simulink model "combinedmodels"  (R2022b)
settings: Solver=VariableStepAuto  StartTime=0.0  StopTime=3600  RelTol=1e-3
libraries: sh_lib x46, spsThreePhaseVIMeasurementLib x36, spsThreePhaseSeriesRLCLoadLib x32, spsThreePhaseSeriesRLCBranchLib x32, fl_lib x27, nesl_utility x25, spsCurrentVoltageSimscapeInterfacegndLib x6, ee_lib x3, spsGroundLib x3, spsPower3phPhasorLib x3, SignalEditorBlockLib x3, spsThreePhaseParallelRLCBranchLib x3
(part 3 of 3)

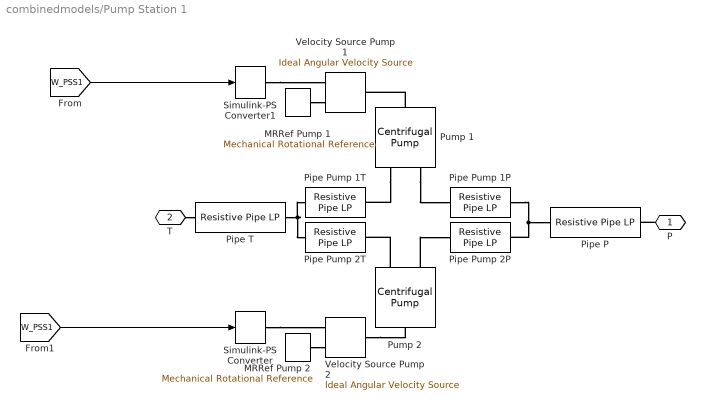
== system combinedmodels/Pump Station 1 ==
  MRRef Pump 1 : fl_lib/Mechanical/Rotational Elements/Mechanical Rotational Reference
  MRRef Pump 2 : fl_lib/Mechanical/Rotational Elements/Mechanical Rotational Reference
  Pipe P : sh_lib/Low-Pressure Blocks/Resistive Pipe LP  cs_type=1  d_in=station_1.pipe_diameter mm  area=1e-04 m^2  D_h=0.0112 m  s_factor=64  length=station_1.pipe_length_3 m  length_ad=1 m  roughness=0.005 mm  Re_lam=2e+03  Re_turb=4e+03  elevation_A=station_1.elevation m  elevation_B=station_1.elevation m  g=9.80665 m/s^2  pressure_drop_specify=off  pressure_drop_priority=None  pressure_drop=0 Pa  pressure_drop_nominal_specify=off  pressure_drop_nominal_unit=Pa  pressure_drop_nominal_value=1  flow_rate_specify=off  flow_rate_priority=None  flow_rate=0 m^3/s  flow_rate_nominal_specify=off  flow_rate_nominal_unit=m^3/s  flow_rate_nominal_value=1
      settings: InternalSimscapePortConfiguration="{\"Bottom\":[],\"Left\":[{\"id\":\"A\",\"label\":\"A\",\"type\":\"foundation.hydraulic.hydraulic\"}],\"Right\":[{\"id\":\"B\",\"label\":\"B\",\"type\":\"foundation.hydraulic.hydraulic\"}],\"Top\":[]}"
  Pipe Pump 1P : sh_lib/Low-Pressure Blocks/Resistive Pipe LP  cs_type=1  d_in=station_1.pipe_diameter mm  area=1e-04 m^2  D_h=0.0112 m  s_factor=64  length=station_1.pipe_length_2 m  length_ad=1 m  roughness=0.005 mm  Re_lam=2e+03  Re_turb=4e+03  elevation_A=station_1.elevation m  elevation_B=station_1.elevation m  g=9.80665 m/s^2  pressure_drop_specify=off  pressure_drop_priority=None  pressure_drop=0 Pa  pressure_drop_nominal_specify=off  pressure_drop_nominal_unit=Pa  pressure_drop_nominal_value=1  flow_rate_specify=off  flow_rate_priority=None  flow_rate=0 m^3/s  flow_rate_nominal_specify=off  flow_rate_nominal_unit=m^3/s  flow_rate_nominal_value=1
      settings: InternalSimscapePortConfiguration="{\"Bottom\":[],\"Left\":[{\"id\":\"A\",\"label\":\"A\",\"type\":\"foundation.hydraulic.hydraulic\"}],\"Right\":[{\"id\":\"B\",\"label\":\"B\",\"type\":\"foundation.hydraulic.hydraulic\"}],\"Top\":[]}"
  Pipe Pump 1T : sh_lib/Low-Pressure Blocks/Resistive Pipe LP  cs_type=1  d_in=station_1.pipe_diameter mm  area=1e-04 m^2  D_h=0.0112 m  s_factor=64  length=station_1.pipe_length_2 m  length_ad=1 m  roughness=0.005 mm  Re_lam=2e+03  Re_turb=4e+03  elevation_A=station_1.elevation m  elevation_B=station_1.elevation m  g=9.80665 m/s^2  pressure_drop_specify=off  pressure_drop_priority=None  pressure_drop=0 Pa  pressure_drop_nominal_specify=off  pressure_drop_nominal_unit=Pa  pressure_drop_nominal_value=1  flow_rate_specify=off  flow_rate_priority=None  flow_rate=0 m^3/s  flow_rate_nominal_specify=off  flow_rate_nominal_unit=m^3/s  flow_rate_nominal_value=1
      settings: InternalSimscapePortConfiguration="{\"Bottom\":[],\"Left\":[{\"id\":\"A\",\"label\":\"A\",\"type\":\"foundation.hydraulic.hydraulic\"}],\"Right\":[{\"id\":\"B\",\"label\":\"B\",\"type\":\"foundation.hydraulic.hydraulic\"}],\"Top\":[]}"
  Pipe Pump 2P : sh_lib/Low-Pressure Blocks/Resistive Pipe LP  cs_type=1  d_in=station_1.pipe_diameter mm  area=1e-04 m^2  D_h=0.0112 m  s_factor=64  length=station_1.pipe_length_2 m  length_ad=1 m  roughness=0.005 mm  Re_lam=2e+03  Re_turb=4e+03  elevation_A=station_1.elevation m  elevation_B=station_1.elevation m  g=9.80665 m/s^2  pressure_drop_specify=off  pressure_drop_priority=None  pressure_drop=0 Pa  pressure_drop_nominal_specify=off  pressure_drop_nominal_unit=Pa  pressure_drop_nominal_value=1  flow_rate_specify=off  flow_rate_priority=None  flow_rate=0 m^3/s  flow_rate_nominal_specify=off  flow_rate_nominal_unit=m^3/s  flow_rate_nominal_value=1
      settings: InternalSimscapePortConfiguration="{\"Bottom\":[],\"Left\":[{\"id\":\"A\",\"label\":\"A\",\"type\":\"foundation.hydraulic.hydraulic\"}],\"Right\":[{\"id\":\"B\",\"label\":\"B\",\"type\":\"foundation.hydraulic.hydraulic\"}],\"Top\":[]}"
  Pipe Pump 2T : sh_lib/Low-Pressure Blocks/Resistive Pipe LP  cs_type=1  d_in=station_1.pipe_diameter mm  area=1e-04 m^2  D_h=0.0112 m  s_factor=64  length=station_1.pipe_length_2 m  length_ad=1 m  roughness=0.005 mm  Re_lam=2e+03  Re_turb=4e+03  elevation_A=station_1.elevation m  elevation_B=station_1.elevation m  g=9.80665 m/s^2  pressure_drop_specify=off  pressure_drop_priority=None  pressure_drop=0 Pa  pressure_drop_nominal_specify=off  pressure_drop_nominal_unit=Pa  pressure_drop_nominal_value=1  flow_rate_specify=off  flow_rate_priority=None  flow_rate=0 m^3/s  flow_rate_nominal_specify=off  flow_rate_nominal_unit=m^3/s  flow_rate_nominal_value=1
      settings: InternalSimscapePortConfiguration="{\"Bottom\":[],\"Left\":[{\"id\":\"A\",\"label\":\"A\",\"type\":\"foundation.hydraulic.hydraulic\"}],\"Right\":[{\"id\":\"B\",\"label\":\"B\",\"type\":\"foundation.hydraulic.hydraulic\"}],\"Top\":[]}"
  Pipe T : sh_lib/Low-Pressure Blocks/Resistive Pipe LP  cs_type=1  d_in=station_1.pipe_diameter mm  area=1e-04 m^2  D_h=0.0112 m  s_factor=64  length=station_1.pipe_length_1 m  length_ad=1 m  roughness=0.005 mm  Re_lam=2e+03  Re_turb=4e+03  elevation_A=station_1.elevation m  elevation_B=station_1.elevation m  g=9.80665 m/s^2  pressure_drop_specify=off  pressure_drop_priority=None  pressure_drop=0 Pa  pressure_drop_nominal_specify=off  pressure_drop_nominal_unit=Pa  pressure_drop_nominal_value=1  flow_rate_specify=off  flow_rate_priority=None  flow_rate=0 m^3/s  flow_rate_nominal_specify=off  flow_rate_nominal_unit=m^3/s  flow_rate_nominal_value=1
      settings: InternalSimscapePortConfiguration="{\"Bottom\":[],\"Left\":[{\"id\":\"A\",\"label\":\"A\",\"type\":\"foundation.hydraulic.hydraulic\"}],\"Right\":[{\"id\":\"B\",\"label\":\"B\",\"type\":\"foundation.hydraulic.hydraulic\"}],\"Top\":[]}"
  Pump 1 : sh_lib/Pumps and Motors/Centrifugal Pump  mdl_type=2  c_1=326.8 Pa/(kg/m^3)  c_2=3.104e+04 Pa*s/kg  c_3=1.097e+07 Pa*s^2/(kg*m^3)  c_4=2.136e+05 Pa*s^2/(kg*m^3)  c_f=0.8  design_del=130 lpm  ref_velocity=2.5e+03 rpm  ref_density=1000 kg/m^3  leak_resistance=1e+8 Pa/(m^3/s)  T_const=0.1 N*m  trq_press_coeff=1e-6 N*m/Pa  pump_del_1D=pump_1.Q m^3/s  press_diff_1D=pump_1.P bar  pump_del_power_1D=pump_1.Q m^3/s  power_1D=pump_1.N W  pump_vel_2D="[  3.2e+03 3.3e+03 3.4e+03 3.5e+03 ] rpm"  pump_del_2D="[  0 50 100 150 200 250 300 350 ] lpm"  press_diff_2D="[  8.3 8.8 9.3 9.9 ; 7.8 8.3 8.8 9.4 ; 7.2 7.6 8.2 8.7 ; 6.5 7 7.5 8 ; 5.6 6.1 6.6 7.1 ; 4.7 5.2 5.7 6.2 ; 3.4 4 4.4 4.9 ; 2.3 2.7 3.4 3.6 ; ] bar"  pump_del_power_2D="[  0 50 100 150 200 250 300 350 ] lpm"  power_2D="[  1.223e+03 1.341e+03 1.467e+03 1.6e+03 ; 1.414e+03 1.551e+03 1.696e+03 1.85e+03 ; 1.636e+03 1.794e+03 1.962e+03 2.14e+03 ; 1.941e+03 2.129e+03 2.326e+03 2.54e+03 ; 2.224e+03 2.439e+03 2.66e+03 2.91e+03 ; 2.453e+03 2.691e+03 2.947e+03 3.21e+03 ; 2.757e+03 3.024e+03 3.307e+03 3.608e+03 ; 2.945e+03 3.23e+03 3.533e+03 3.854e+03 ; ] W"  omega_threshold=1e-9 rad/s  interp_method=2  extrap_method=1
      settings: InternalSimscapePortConfiguration="{\"Bottom\":[],\"Left\":[{\"id\":\"S\",\"label\":\"S\",\"type\":\"foundation.mechanical.rotational.rotational\"}],\"Right\":[{\"id\":\"P\",\"label\":\"P\",\"type\":\"foundation.hydraulic.hydraulic\"},{\"id\":\"T\",\"label\":\"T\",\"type\":\"foundation.hydraulic.hydraulic\"}],\"Top\":[]}"
  Pump 2 : sh_lib/Pumps and Motors/Centrifugal Pump  mdl_type=2  c_1=326.8 Pa/(kg/m^3)  c_2=3.104e+04 Pa*s/kg  c_3=1.097e+07 Pa*s^2/(kg*m^3)  c_4=2.136e+05 Pa*s^2/(kg*m^3)  c_f=0.8  design_del=130 lpm  ref_velocity=2.5e+03 rpm  ref_density=1000 kg/m^3  leak_resistance=1e+8 Pa/(m^3/s)  T_const=0.1 N*m  trq_press_coeff=1e-6 N*m/Pa  pump_del_1D=pump_1.Q m^3/s  press_diff_1D=pump_1.P bar  pump_del_power_1D=pump_1.Q m^3/s  power_1D=pump_1.N W  pump_vel_2D="[  3.2e+03 3.3e+03 3.4e+03 3.5e+03 ] rpm"  pump_del_2D="[  0 50 100 150 200 250 300 350 ] lpm"  press_diff_2D="[  8.3 8.8 9.3 9.9 ; 7.8 8.3 8.8 9.4 ; 7.2 7.6 8.2 8.7 ; 6.5 7 7.5 8 ; 5.6 6.1 6.6 7.1 ; 4.7 5.2 5.7 6.2 ; 3.4 4 4.4 4.9 ; 2.3 2.7 3.4 3.6 ; ] bar"  pump_del_power_2D="[  0 50 100 150 200 250 300 350 ] lpm"  power_2D="[  1.223e+03 1.341e+03 1.467e+03 1.6e+03 ; 1.414e+03 1.551e+03 1.696e+03 1.85e+03 ; 1.636e+03 1.794e+03 1.962e+03 2.14e+03 ; 1.941e+03 2.129e+03 2.326e+03 2.54e+03 ; 2.224e+03 2.439e+03 2.66e+03 2.91e+03 ; 2.453e+03 2.691e+03 2.947e+03 3.21e+03 ; 2.757e+03 3.024e+03 3.307e+03 3.608e+03 ; 2.945e+03 3.23e+03 3.533e+03 3.854e+03 ; ] W"  omega_threshold=1e-9 rad/s  interp_method=2  extrap_method=1
      settings: InternalSimscapePortConfiguration="{\"Bottom\":[],\"Left\":[{\"id\":\"S\",\"label\":\"S\",\"type\":\"foundation.mechanical.rotational.rotational\"}],\"Right\":[{\"id\":\"P\",\"label\":\"P\",\"type\":\"foundation.hydraulic.hydraulic\"},{\"id\":\"T\",\"label\":\"T\",\"type\":\"foundation.hydraulic.hydraulic\"}],\"Top\":[]}"
  Simulink-PS Converter : nesl_utility/Simulink-PS Converter  PhysicalDomain=network_engine_domain  SubClassName=ps_input  LeftPortType=input  RightPortType=output  PseudoPeriodic=off  Frequencies=[]  NoiseDistribution=none  NoiseParameters=[]  Unit=rpm  AffineConversion=off  FilteringAndDerivatives=zero  SimscapeFilterOrder=1  InputFilterTimeConstant=.001  UdotUserProvided=0
  Simulink-PS Converter1 : nesl_utility/Simulink-PS Converter  PhysicalDomain=network_engine_domain  SubClassName=ps_input  LeftPortType=input  RightPortType=output  PseudoPeriodic=off  Frequencies=[]  NoiseDistribution=none  NoiseParameters=[]  Unit=rpm  AffineConversion=off  FilteringAndDerivatives=zero  SimscapeFilterOrder=1  InputFilterTimeConstant=.001  UdotUserProvided=0
  Velocity Source Pump 1 : fl_lib/Mechanical/Mechanical Sources/Ideal Angular Velocity Source
  Velocity Source Pump 2 : fl_lib/Mechanical/Mechanical Sources/Ideal Angular Velocity Source
  P : PMIOPort  Side=Right
  T : PMIOPort  Port=2  Side=Left
  wires:
  [W_PSS1] -> Simulink-PS Converter/1
  [W_PSS1] -> Simulink-PS Converter1/1
  connections:
  Velocity Source Pump 2/LConn1 -- Pump 2/LConn1
  Pump 1/RConn1 -- Pipe Pump 1P/LConn1
  Pump 1/RConn2 -- Pipe Pump 1T/RConn1
  Pump 2/RConn2 -- Pipe Pump 2T/RConn1
  T/RConn1 -- Pipe T/LConn1
  Pump 2/RConn1 -- Pipe Pump 2P/LConn1
  Pipe T/RConn1 -- Pipe Pump 2T/LConn1 -- Pipe Pump 1T/LConn1
  Simulink-PS Converter/RConn1 -- Velocity Source Pump 2/RConn1
  MRRef Pump 2/LConn1 -- Velocity Source Pump 2/RConn2
  Pipe Pump 1P/RConn1 -- Pipe Pump 2P/RConn1 -- Pipe P/LConn1
  P/RConn1 -- Pipe P/RConn1
  MRRef Pump 1/LConn1 -- Velocity Source Pump 1/RConn2
  Pump 1/LConn1 -- Velocity Source Pump 1/LConn1
  Simulink-PS Converter1/RConn1 -- Velocity Source Pump 1/RConn1

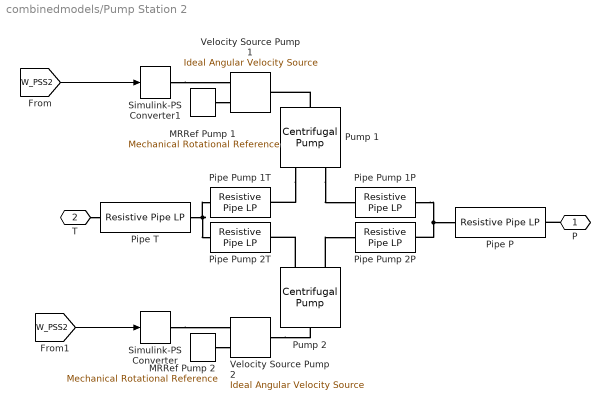
== system combinedmodels/Pump Station 2 ==
  MRRef Pump 1 : fl_lib/Mechanical/Rotational Elements/Mechanical Rotational Reference
  MRRef Pump 2 : fl_lib/Mechanical/Rotational Elements/Mechanical Rotational Reference
  Pipe P : sh_lib/Low-Pressure Blocks/Resistive Pipe LP  cs_type=1  d_in=station_1.pipe_diameter mm  area=1e-04 m^2  D_h=0.0112 m  s_factor=64  length=station_1.pipe_length_3 m  length_ad=1 m  roughness=0.005 mm  Re_lam=2e+03  Re_turb=4e+03  elevation_A=station_1.elevation m  elevation_B=station_1.elevation m  g=9.80665 m/s^2  pressure_drop_specify=off  pressure_drop_priority=None  pressure_drop=0 Pa  pressure_drop_nominal_specify=off  pressure_drop_nominal_unit=Pa  pressure_drop_nominal_value=1  flow_rate_specify=off  flow_rate_priority=None  flow_rate=0 m^3/s  flow_rate_nominal_specify=off  flow_rate_nominal_unit=m^3/s  flow_rate_nominal_value=1
      settings: InternalSimscapePortConfiguration="{\"Bottom\":[],\"Left\":[{\"id\":\"A\",\"label\":\"A\",\"type\":\"foundation.hydraulic.hydraulic\"}],\"Right\":[{\"id\":\"B\",\"label\":\"B\",\"type\":\"foundation.hydraulic.hydraulic\"}],\"Top\":[]}"
  Pipe Pump 1P : sh_lib/Low-Pressure Blocks/Resistive Pipe LP  cs_type=1  d_in=station_1.pipe_diameter mm  area=1e-04 m^2  D_h=0.0112 m  s_factor=64  length=station_1.pipe_length_2 m  length_ad=1 m  roughness=0.005 mm  Re_lam=2e+03  Re_turb=4e+03  elevation_A=station_1.elevation m  elevation_B=station_1.elevation m  g=9.80665 m/s^2  pressure_drop_specify=off  pressure_drop_priority=None  pressure_drop=0 Pa  pressure_drop_nominal_specify=off  pressure_drop_nominal_unit=Pa  pressure_drop_nominal_value=1  flow_rate_specify=off  flow_rate_priority=None  flow_rate=0 m^3/s  flow_rate_nominal_specify=off  flow_rate_nominal_unit=m^3/s  flow_rate_nominal_value=1
      settings: InternalSimscapePortConfiguration="{\"Bottom\":[],\"Left\":[{\"id\":\"A\",\"label\":\"A\",\"type\":\"foundation.hydraulic.hydraulic\"}],\"Right\":[{\"id\":\"B\",\"label\":\"B\",\"type\":\"foundation.hydraulic.hydraulic\"}],\"Top\":[]}"
  Pipe Pump 1T : sh_lib/Low-Pressure Blocks/Resistive Pipe LP  cs_type=1  d_in=station_1.pipe_diameter mm  area=1e-04 m^2  D_h=0.0112 m  s_factor=64  length=station_1.pipe_length_2 m  length_ad=1 m  roughness=0.005 mm  Re_lam=2e+03  Re_turb=4e+03  elevation_A=station_1.elevation m  elevation_B=station_1.elevation m  g=9.80665 m/s^2  pressure_drop_specify=off  pressure_drop_priority=None  pressure_drop=0 Pa  pressure_drop_nominal_specify=off  pressure_drop_nominal_unit=Pa  pressure_drop_nominal_value=1  flow_rate_specify=off  flow_rate_priority=None  flow_rate=0 m^3/s  flow_rate_nominal_specify=off  flow_rate_nominal_unit=m^3/s  flow_rate_nominal_value=1
      settings: InternalSimscapePortConfiguration="{\"Bottom\":[],\"Left\":[{\"id\":\"A\",\"label\":\"A\",\"type\":\"foundation.hydraulic.hydraulic\"}],\"Right\":[{\"id\":\"B\",\"label\":\"B\",\"type\":\"foundation.hydraulic.hydraulic\"}],\"Top\":[]}"
  Pipe Pump 2P : sh_lib/Low-Pressure Blocks/Resistive Pipe LP  cs_type=1  d_in=station_1.pipe_diameter mm  area=1e-04 m^2  D_h=0.0112 m  s_factor=64  length=station_1.pipe_length_2 m  length_ad=1 m  roughness=0.005 mm  Re_lam=2e+03  Re_turb=4e+03  elevation_A=station_1.elevation m  elevation_B=station_1.elevation m  g=9.80665 m/s^2  pressure_drop_specify=off  pressure_drop_priority=None  pressure_drop=0 Pa  pressure_drop_nominal_specify=off  pressure_drop_nominal_unit=Pa  pressure_drop_nominal_value=1  flow_rate_specify=off  flow_rate_priority=None  flow_rate=0 m^3/s  flow_rate_nominal_specify=off  flow_rate_nominal_unit=m^3/s  flow_rate_nominal_value=1
      settings: InternalSimscapePortConfiguration="{\"Bottom\":[],\"Left\":[{\"id\":\"A\",\"label\":\"A\",\"type\":\"foundation.hydraulic.hydraulic\"}],\"Right\":[{\"id\":\"B\",\"label\":\"B\",\"type\":\"foundation.hydraulic.hydraulic\"}],\"Top\":[]}"
  Pipe Pump 2T : sh_lib/Low-Pressure Blocks/Resistive Pipe LP  cs_type=1  d_in=station_1.pipe_diameter mm  area=1e-04 m^2  D_h=0.0112 m  s_factor=64  length=station_1.pipe_length_2 m  length_ad=1 m  roughness=0.005 mm  Re_lam=2e+03  Re_turb=4e+03  elevation_A=station_1.elevation m  elevation_B=station_1.elevation m  g=9.80665 m/s^2  pressure_drop_specify=off  pressure_drop_priority=None  pressure_drop=0 Pa  pressure_drop_nominal_specify=off  pressure_drop_nominal_unit=Pa  pressure_drop_nominal_value=1  flow_rate_specify=off  flow_rate_priority=None  flow_rate=0 m^3/s  flow_rate_nominal_specify=off  flow_rate_nominal_unit=m^3/s  flow_rate_nominal_value=1
      settings: InternalSimscapePortConfiguration="{\"Bottom\":[],\"Left\":[{\"id\":\"A\",\"label\":\"A\",\"type\":\"foundation.hydraulic.hydraulic\"}],\"Right\":[{\"id\":\"B\",\"label\":\"B\",\"type\":\"foundation.hydraulic.hydraulic\"}],\"Top\":[]}"
  Pipe T : sh_lib/Low-Pressure Blocks/Resistive Pipe LP  cs_type=1  d_in=station_1.pipe_diameter mm  area=1e-04 m^2  D_h=0.0112 m  s_factor=64  length=station_1.pipe_length_1 m  length_ad=1 m  roughness=0.005 mm  Re_lam=2e+03  Re_turb=4e+03  elevation_A=station_1.elevation m  elevation_B=station_1.elevation m  g=9.80665 m/s^2  pressure_drop_specify=off  pressure_drop_priority=None  pressure_drop=0 Pa  pressure_drop_nominal_specify=off  pressure_drop_nominal_unit=Pa  pressure_drop_nominal_value=1  flow_rate_specify=off  flow_rate_priority=None  flow_rate=0 m^3/s  flow_rate_nominal_specify=off  flow_rate_nominal_unit=m^3/s  flow_rate_nominal_value=1
      settings: InternalSimscapePortConfiguration="{\"Bottom\":[],\"Left\":[{\"id\":\"A\",\"label\":\"A\",\"type\":\"foundation.hydraulic.hydraulic\"}],\"Right\":[{\"id\":\"B\",\"label\":\"B\",\"type\":\"foundation.hydraulic.hydraulic\"}],\"Top\":[]}"
  Pump 1 : sh_lib/Pumps and Motors/Centrifugal Pump  mdl_type=2  c_1=326.8 Pa/(kg/m^3)  c_2=3.104e+04 Pa*s/kg  c_3=1.097e+07 Pa*s^2/(kg*m^3)  c_4=2.136e+05 Pa*s^2/(kg*m^3)  c_f=0.8  design_del=130 lpm  ref_velocity=2.5e+03 rpm  ref_density=1000 kg/m^3  leak_resistance=1e+8 Pa/(m^3/s)  T_const=0.1 N*m  trq_press_coeff=1e-6 N*m/Pa  pump_del_1D=pump_1.Q m^3/s  press_diff_1D=pump_1.P bar  pump_del_power_1D=pump_1.Q m^3/s  power_1D=pump_1.N W  pump_vel_2D="[  3.2e+03 3.3e+03 3.4e+03 3.5e+03 ] rpm"  pump_del_2D="[  0 50 100 150 200 250 300 350 ] lpm"  press_diff_2D="[  8.3 8.8 9.3 9.9 ; 7.8 8.3 8.8 9.4 ; 7.2 7.6 8.2 8.7 ; 6.5 7 7.5 8 ; 5.6 6.1 6.6 7.1 ; 4.7 5.2 5.7 6.2 ; 3.4 4 4.4 4.9 ; 2.3 2.7 3.4 3.6 ; ] bar"  pump_del_power_2D="[  0 50 100 150 200 250 300 350 ] lpm"  power_2D="[  1.223e+03 1.341e+03 1.467e+03 1.6e+03 ; 1.414e+03 1.551e+03 1.696e+03 1.85e+03 ; 1.636e+03 1.794e+03 1.962e+03 2.14e+03 ; 1.941e+03 2.129e+03 2.326e+03 2.54e+03 ; 2.224e+03 2.439e+03 2.66e+03 2.91e+03 ; 2.453e+03 2.691e+03 2.947e+03 3.21e+03 ; 2.757e+03 3.024e+03 3.307e+03 3.608e+03 ; 2.945e+03 3.23e+03 3.533e+03 3.854e+03 ; ] W"  omega_threshold=1e-9 rad/s  interp_method=2  extrap_method=1
      settings: InternalSimscapePortConfiguration="{\"Bottom\":[],\"Left\":[{\"id\":\"S\",\"label\":\"S\",\"type\":\"foundation.mechanical.rotational.rotational\"}],\"Right\":[{\"id\":\"P\",\"label\":\"P\",\"type\":\"foundation.hydraulic.hydraulic\"},{\"id\":\"T\",\"label\":\"T\",\"type\":\"foundation.hydraulic.hydraulic\"}],\"Top\":[]}"
  Pump 2 : sh_lib/Pumps and Motors/Centrifugal Pump  mdl_type=2  c_1=326.8 Pa/(kg/m^3)  c_2=3.104e+04 Pa*s/kg  c_3=1.097e+07 Pa*s^2/(kg*m^3)  c_4=2.136e+05 Pa*s^2/(kg*m^3)  c_f=0.8  design_del=130 lpm  ref_velocity=2.5e+03 rpm  ref_density=1000 kg/m^3  leak_resistance=1e+8 Pa/(m^3/s)  T_const=0.1 N*m  trq_press_coeff=1e-6 N*m/Pa  pump_del_1D=pump_1.Q m^3/s  press_diff_1D=pump_1.P bar  pump_del_power_1D=pump_1.Q m^3/s  power_1D=pump_1.N W  pump_vel_2D="[  3.2e+03 3.3e+03 3.4e+03 3.5e+03 ] rpm"  pump_del_2D="[  0 50 100 150 200 250 300 350 ] lpm"  press_diff_2D="[  8.3 8.8 9.3 9.9 ; 7.8 8.3 8.8 9.4 ; 7.2 7.6 8.2 8.7 ; 6.5 7 7.5 8 ; 5.6 6.1 6.6 7.1 ; 4.7 5.2 5.7 6.2 ; 3.4 4 4.4 4.9 ; 2.3 2.7 3.4 3.6 ; ] bar"  pump_del_power_2D="[  0 50 100 150 200 250 300 350 ] lpm"  power_2D="[  1.223e+03 1.341e+03 1.467e+03 1.6e+03 ; 1.414e+03 1.551e+03 1.696e+03 1.85e+03 ; 1.636e+03 1.794e+03 1.962e+03 2.14e+03 ; 1.941e+03 2.129e+03 2.326e+03 2.54e+03 ; 2.224e+03 2.439e+03 2.66e+03 2.91e+03 ; 2.453e+03 2.691e+03 2.947e+03 3.21e+03 ; 2.757e+03 3.024e+03 3.307e+03 3.608e+03 ; 2.945e+03 3.23e+03 3.533e+03 3.854e+03 ; ] W"  omega_threshold=1e-9 rad/s  interp_method=2  extrap_method=1
      settings: InternalSimscapePortConfiguration="{\"Bottom\":[],\"Left\":[{\"id\":\"S\",\"label\":\"S\",\"type\":\"foundation.mechanical.rotational.rotational\"}],\"Right\":[{\"id\":\"P\",\"label\":\"P\",\"type\":\"foundation.hydraulic.hydraulic\"},{\"id\":\"T\",\"label\":\"T\",\"type\":\"foundation.hydraulic.hydraulic\"}],\"Top\":[]}"
  Simulink-PS Converter : nesl_utility/Simulink-PS Converter  PhysicalDomain=network_engine_domain  SubClassName=ps_input  LeftPortType=input  RightPortType=output  PseudoPeriodic=off  Frequencies=[]  NoiseDistribution=none  NoiseParameters=[]  Unit=rpm  AffineConversion=off  FilteringAndDerivatives=zero  SimscapeFilterOrder=1  InputFilterTimeConstant=.001  UdotUserProvided=0
  Simulink-PS Converter1 : nesl_utility/Simulink-PS Converter  PhysicalDomain=network_engine_domain  SubClassName=ps_input  LeftPortType=input  RightPortType=output  PseudoPeriodic=off  Frequencies=[]  NoiseDistribution=none  NoiseParameters=[]  Unit=rpm  AffineConversion=off  FilteringAndDerivatives=zero  SimscapeFilterOrder=1  InputFilterTimeConstant=.001  UdotUserProvided=0
  Velocity Source Pump 1 : fl_lib/Mechanical/Mechanical Sources/Ideal Angular Velocity Source
  Velocity Source Pump 2 : fl_lib/Mechanical/Mechanical Sources/Ideal Angular Velocity Source
  P : PMIOPort  Side=Right
  T : PMIOPort  Port=2  Side=Left
  wires:
  [W_PSS2] -> Simulink-PS Converter/1
  [W_PSS2] -> Simulink-PS Converter1/1
  connections:
  Velocity Source Pump 2/LConn1 -- Pump 2/LConn1
  Pump 1/RConn1 -- Pipe Pump 1P/LConn1
  Pump 1/RConn2 -- Pipe Pump 1T/RConn1
  Pump 2/RConn2 -- Pipe Pump 2T/RConn1
  T/RConn1 -- Pipe T/LConn1
  Pump 2/RConn1 -- Pipe Pump 2P/LConn1
  Pipe T/RConn1 -- Pipe Pump 2T/LConn1 -- Pipe Pump 1T/LConn1
  Simulink-PS Converter/RConn1 -- Velocity Source Pump 2/RConn1
  MRRef Pump 2/LConn1 -- Velocity Source Pump 2/RConn2
  Pipe Pump 1P/RConn1 -- Pipe Pump 2P/RConn1 -- Pipe P/LConn1
  P/RConn1 -- Pipe P/RConn1
  MRRef Pump 1/LConn1 -- Velocity Source Pump 1/RConn2
  Pump 1/LConn1 -- Velocity Source Pump 1/LConn1
  Simulink-PS Converter1/RConn1 -- Velocity Source Pump 1/RConn1

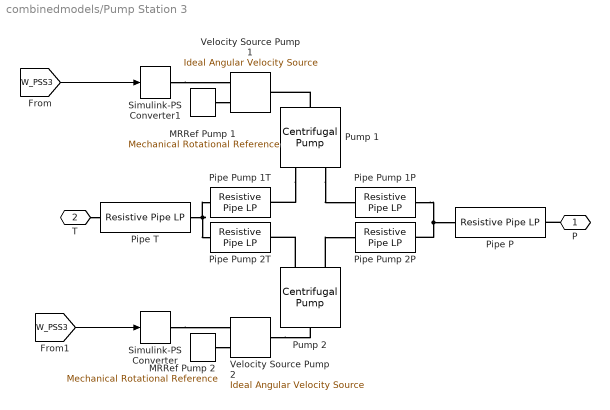
== system combinedmodels/Pump Station 3 ==
  MRRef Pump 1 : fl_lib/Mechanical/Rotational Elements/Mechanical Rotational Reference
  MRRef Pump 2 : fl_lib/Mechanical/Rotational Elements/Mechanical Rotational Reference
  Pipe P : sh_lib/Low-Pressure Blocks/Resistive Pipe LP  cs_type=1  d_in=station_1.pipe_diameter mm  area=1e-04 m^2  D_h=0.0112 m  s_factor=64  length=station_1.pipe_length_3 m  length_ad=1 m  roughness=0.005 mm  Re_lam=2e+03  Re_turb=4e+03  elevation_A=station_1.elevation m  elevation_B=station_1.elevation m  g=9.80665 m/s^2  pressure_drop_specify=off  pressure_drop_priority=None  pressure_drop=0 Pa  pressure_drop_nominal_specify=off  pressure_drop_nominal_unit=Pa  pressure_drop_nominal_value=1  flow_rate_specify=off  flow_rate_priority=None  flow_rate=0 m^3/s  flow_rate_nominal_specify=off  flow_rate_nominal_unit=m^3/s  flow_rate_nominal_value=1
      settings: InternalSimscapePortConfiguration="{\"Bottom\":[],\"Left\":[{\"id\":\"A\",\"label\":\"A\",\"type\":\"foundation.hydraulic.hydraulic\"}],\"Right\":[{\"id\":\"B\",\"label\":\"B\",\"type\":\"foundation.hydraulic.hydraulic\"}],\"Top\":[]}"
  Pipe Pump 1P : sh_lib/Low-Pressure Blocks/Resistive Pipe LP  cs_type=1  d_in=station_1.pipe_diameter mm  area=1e-04 m^2  D_h=0.0112 m  s_factor=64  length=station_1.pipe_length_2 m  length_ad=1 m  roughness=0.005 mm  Re_lam=2e+03  Re_turb=4e+03  elevation_A=station_1.elevation m  elevation_B=station_1.elevation m  g=9.80665 m/s^2  pressure_drop_specify=off  pressure_drop_priority=None  pressure_drop=0 Pa  pressure_drop_nominal_specify=off  pressure_drop_nominal_unit=Pa  pressure_drop_nominal_value=1  flow_rate_specify=off  flow_rate_priority=None  flow_rate=0 m^3/s  flow_rate_nominal_specify=off  flow_rate_nominal_unit=m^3/s  flow_rate_nominal_value=1
      settings: InternalSimscapePortConfiguration="{\"Bottom\":[],\"Left\":[{\"id\":\"A\",\"label\":\"A\",\"type\":\"foundation.hydraulic.hydraulic\"}],\"Right\":[{\"id\":\"B\",\"label\":\"B\",\"type\":\"foundation.hydraulic.hydraulic\"}],\"Top\":[]}"
  Pipe Pump 1T : sh_lib/Low-Pressure Blocks/Resistive Pipe LP  cs_type=1  d_in=station_1.pipe_diameter mm  area=1e-04 m^2  D_h=0.0112 m  s_factor=64  length=station_1.pipe_length_2 m  length_ad=1 m  roughness=0.005 mm  Re_lam=2e+03  Re_turb=4e+03  elevation_A=station_1.elevation m  elevation_B=station_1.elevation m  g=9.80665 m/s^2  pressure_drop_specify=off  pressure_drop_priority=None  pressure_drop=0 Pa  pressure_drop_nominal_specify=off  pressure_drop_nominal_unit=Pa  pressure_drop_nominal_value=1  flow_rate_specify=off  flow_rate_priority=None  flow_rate=0 m^3/s  flow_rate_nominal_specify=off  flow_rate_nominal_unit=m^3/s  flow_rate_nominal_value=1
      settings: InternalSimscapePortConfiguration="{\"Bottom\":[],\"Left\":[{\"id\":\"A\",\"label\":\"A\",\"type\":\"foundation.hydraulic.hydraulic\"}],\"Right\":[{\"id\":\"B\",\"label\":\"B\",\"type\":\"foundation.hydraulic.hydraulic\"}],\"Top\":[]}"
  Pipe Pump 2P : sh_lib/Low-Pressure Blocks/Resistive Pipe LP  cs_type=1  d_in=station_1.pipe_diameter mm  area=1e-04 m^2  D_h=0.0112 m  s_factor=64  length=station_1.pipe_length_2 m  length_ad=1 m  roughness=0.005 mm  Re_lam=2e+03  Re_turb=4e+03  elevation_A=station_1.elevation m  elevation_B=station_1.elevation m  g=9.80665 m/s^2  pressure_drop_specify=off  pressure_drop_priority=None  pressure_drop=0 Pa  pressure_drop_nominal_specify=off  pressure_drop_nominal_unit=Pa  pressure_drop_nominal_value=1  flow_rate_specify=off  flow_rate_priority=None  flow_rate=0 m^3/s  flow_rate_nominal_specify=off  flow_rate_nominal_unit=m^3/s  flow_rate_nominal_value=1
      settings: InternalSimscapePortConfiguration="{\"Bottom\":[],\"Left\":[{\"id\":\"A\",\"label\":\"A\",\"type\":\"foundation.hydraulic.hydraulic\"}],\"Right\":[{\"id\":\"B\",\"label\":\"B\",\"type\":\"foundation.hydraulic.hydraulic\"}],\"Top\":[]}"
  Pipe Pump 2T : sh_lib/Low-Pressure Blocks/Resistive Pipe LP  cs_type=1  d_in=station_1.pipe_diameter mm  area=1e-04 m^2  D_h=0.0112 m  s_factor=64  length=station_1.pipe_length_2 m  length_ad=1 m  roughness=0.005 mm  Re_lam=2e+03  Re_turb=4e+03  elevation_A=station_1.elevation m  elevation_B=station_1.elevation m  g=9.80665 m/s^2  pressure_drop_specify=off  pressure_drop_priority=None  pressure_drop=0 Pa  pressure_drop_nominal_specify=off  pressure_drop_nominal_unit=Pa  pressure_drop_nominal_value=1  flow_rate_specify=off  flow_rate_priority=None  flow_rate=0 m^3/s  flow_rate_nominal_specify=off  flow_rate_nominal_unit=m^3/s  flow_rate_nominal_value=1
      settings: InternalSimscapePortConfiguration="{\"Bottom\":[],\"Left\":[{\"id\":\"A\",\"label\":\"A\",\"type\":\"foundation.hydraulic.hydraulic\"}],\"Right\":[{\"id\":\"B\",\"label\":\"B\",\"type\":\"foundation.hydraulic.hydraulic\"}],\"Top\":[]}"
  Pipe T : sh_lib/Low-Pressure Blocks/Resistive Pipe LP  cs_type=1  d_in=station_1.pipe_diameter mm  area=1e-04 m^2  D_h=0.0112 m  s_factor=64  length=station_1.pipe_length_1 m  length_ad=1 m  roughness=0.005 mm  Re_lam=2e+03  Re_turb=4e+03  elevation_A=station_1.elevation m  elevation_B=station_1.elevation m  g=9.80665 m/s^2  pressure_drop_specify=off  pressure_drop_priority=None  pressure_drop=0 Pa  pressure_drop_nominal_specify=off  pressure_drop_nominal_unit=Pa  pressure_drop_nominal_value=1  flow_rate_specify=off  flow_rate_priority=None  flow_rate=0 m^3/s  flow_rate_nominal_specify=off  flow_rate_nominal_unit=m^3/s  flow_rate_nominal_value=1
      settings: InternalSimscapePortConfiguration="{\"Bottom\":[],\"Left\":[{\"id\":\"A\",\"label\":\"A\",\"type\":\"foundation.hydraulic.hydraulic\"}],\"Right\":[{\"id\":\"B\",\"label\":\"B\",\"type\":\"foundation.hydraulic.hydraulic\"}],\"Top\":[]}"
  Pump 1 : sh_lib/Pumps and Motors/Centrifugal Pump  mdl_type=2  c_1=326.8 Pa/(kg/m^3)  c_2=3.104e+04 Pa*s/kg  c_3=1.097e+07 Pa*s^2/(kg*m^3)  c_4=2.136e+05 Pa*s^2/(kg*m^3)  c_f=0.8  design_del=130 lpm  ref_velocity=2.5e+03 rpm  ref_density=1000 kg/m^3  leak_resistance=1e+8 Pa/(m^3/s)  T_const=0.1 N*m  trq_press_coeff=1e-6 N*m/Pa  pump_del_1D=pump_1.Q m^3/s  press_diff_1D=pump_1.P bar  pump_del_power_1D=pump_1.Q m^3/s  power_1D=pump_1.N W  pump_vel_2D="[  3.2e+03 3.3e+03 3.4e+03 3.5e+03 ] rpm"  pump_del_2D="[  0 50 100 150 200 250 300 350 ] lpm"  press_diff_2D="[  8.3 8.8 9.3 9.9 ; 7.8 8.3 8.8 9.4 ; 7.2 7.6 8.2 8.7 ; 6.5 7 7.5 8 ; 5.6 6.1 6.6 7.1 ; 4.7 5.2 5.7 6.2 ; 3.4 4 4.4 4.9 ; 2.3 2.7 3.4 3.6 ; ] bar"  pump_del_power_2D="[  0 50 100 150 200 250 300 350 ] lpm"  power_2D="[  1.223e+03 1.341e+03 1.467e+03 1.6e+03 ; 1.414e+03 1.551e+03 1.696e+03 1.85e+03 ; 1.636e+03 1.794e+03 1.962e+03 2.14e+03 ; 1.941e+03 2.129e+03 2.326e+03 2.54e+03 ; 2.224e+03 2.439e+03 2.66e+03 2.91e+03 ; 2.453e+03 2.691e+03 2.947e+03 3.21e+03 ; 2.757e+03 3.024e+03 3.307e+03 3.608e+03 ; 2.945e+03 3.23e+03 3.533e+03 3.854e+03 ; ] W"  omega_threshold=1e-9 rad/s  interp_method=2  extrap_method=1
      settings: InternalSimscapePortConfiguration="{\"Bottom\":[],\"Left\":[{\"id\":\"S\",\"label\":\"S\",\"type\":\"foundation.mechanical.rotational.rotational\"}],\"Right\":[{\"id\":\"P\",\"label\":\"P\",\"type\":\"foundation.hydraulic.hydraulic\"},{\"id\":\"T\",\"label\":\"T\",\"type\":\"foundation.hydraulic.hydraulic\"}],\"Top\":[]}"
  Pump 2 : sh_lib/Pumps and Motors/Centrifugal Pump  mdl_type=2  c_1=326.8 Pa/(kg/m^3)  c_2=3.104e+04 Pa*s/kg  c_3=1.097e+07 Pa*s^2/(kg*m^3)  c_4=2.136e+05 Pa*s^2/(kg*m^3)  c_f=0.8  design_del=130 lpm  ref_velocity=2.5e+03 rpm  ref_density=1000 kg/m^3  leak_resistance=1e+8 Pa/(m^3/s)  T_const=0.1 N*m  trq_press_coeff=1e-6 N*m/Pa  pump_del_1D=pump_1.Q m^3/s  press_diff_1D=pump_1.P bar  pump_del_power_1D=pump_1.Q m^3/s  power_1D=pump_1.N W  pump_vel_2D="[  3.2e+03 3.3e+03 3.4e+03 3.5e+03 ] rpm"  pump_del_2D="[  0 50 100 150 200 250 300 350 ] lpm"  press_diff_2D="[  8.3 8.8 9.3 9.9 ; 7.8 8.3 8.8 9.4 ; 7.2 7.6 8.2 8.7 ; 6.5 7 7.5 8 ; 5.6 6.1 6.6 7.1 ; 4.7 5.2 5.7 6.2 ; 3.4 4 4.4 4.9 ; 2.3 2.7 3.4 3.6 ; ] bar"  pump_del_power_2D="[  0 50 100 150 200 250 300 350 ] lpm"  power_2D="[  1.223e+03 1.341e+03 1.467e+03 1.6e+03 ; 1.414e+03 1.551e+03 1.696e+03 1.85e+03 ; 1.636e+03 1.794e+03 1.962e+03 2.14e+03 ; 1.941e+03 2.129e+03 2.326e+03 2.54e+03 ; 2.224e+03 2.439e+03 2.66e+03 2.91e+03 ; 2.453e+03 2.691e+03 2.947e+03 3.21e+03 ; 2.757e+03 3.024e+03 3.307e+03 3.608e+03 ; 2.945e+03 3.23e+03 3.533e+03 3.854e+03 ; ] W"  omega_threshold=1e-9 rad/s  interp_method=2  extrap_method=1
      settings: InternalSimscapePortConfiguration="{\"Bottom\":[],\"Left\":[{\"id\":\"S\",\"label\":\"S\",\"type\":\"foundation.mechanical.rotational.rotational\"}],\"Right\":[{\"id\":\"P\",\"label\":\"P\",\"type\":\"foundation.hydraulic.hydraulic\"},{\"id\":\"T\",\"label\":\"T\",\"type\":\"foundation.hydraulic.hydraulic\"}],\"Top\":[]}"
  Simulink-PS Converter : nesl_utility/Simulink-PS Converter  PhysicalDomain=network_engine_domain  SubClassName=ps_input  LeftPortType=input  RightPortType=output  PseudoPeriodic=off  Frequencies=[]  NoiseDistribution=none  NoiseParameters=[]  Unit=rpm  AffineConversion=off  FilteringAndDerivatives=zero  SimscapeFilterOrder=1  InputFilterTimeConstant=.001  UdotUserProvided=0
  Simulink-PS Converter1 : nesl_utility/Simulink-PS Converter  PhysicalDomain=network_engine_domain  SubClassName=ps_input  LeftPortType=input  RightPortType=output  PseudoPeriodic=off  Frequencies=[]  NoiseDistribution=none  NoiseParameters=[]  Unit=rpm  AffineConversion=off  FilteringAndDerivatives=zero  SimscapeFilterOrder=1  InputFilterTimeConstant=.001  UdotUserProvided=0
  Velocity Source Pump 1 : fl_lib/Mechanical/Mechanical Sources/Ideal Angular Velocity Source
  Velocity Source Pump 2 : fl_lib/Mechanical/Mechanical Sources/Ideal Angular Velocity Source
  P : PMIOPort  Side=Right
  T : PMIOPort  Port=2  Side=Left
  wires:
  [W_PSS3] -> Simulink-PS Converter/1
  [W_PSS3] -> Simulink-PS Converter1/1
  connections:
  Velocity Source Pump 2/LConn1 -- Pump 2/LConn1
  Pump 1/RConn1 -- Pipe Pump 1P/LConn1
  Pump 1/RConn2 -- Pipe Pump 1T/RConn1
  Pump 2/RConn2 -- Pipe Pump 2T/RConn1
  T/RConn1 -- Pipe T/LConn1
  Pump 2/RConn1 -- Pipe Pump 2P/LConn1
  Pipe T/RConn1 -- Pipe Pump 2T/LConn1 -- Pipe Pump 1T/LConn1
  Simulink-PS Converter/RConn1 -- Velocity Source Pump 2/RConn1
  MRRef Pump 2/LConn1 -- Velocity Source Pump 2/RConn2
  Pipe Pump 1P/RConn1 -- Pipe Pump 2P/RConn1 -- Pipe P/LConn1
  P/RConn1 -- Pipe P/RConn1
  MRRef Pump 1/LConn1 -- Velocity Source Pump 1/RConn2
  Pump 1/LConn1 -- Velocity Source Pump 1/LConn1
  Simulink-PS Converter1/RConn1 -- Velocity Source Pump 1/RConn1

== system combinedmodels/Subsystem ==
  Flow Control Valve : sh_lib/Valves/Flow Control Valves/Pressure-Compensated Flow Control Valve  Tag=Factory Generic  mdl_type=1  area_max=0.86e-4 m^2  opening_max=0.02 m  opening_tab="[  -0.002 0 0.005 0.015 ] m"  area_tab="[  1e-12 4e-12 1e-05 1.02e-05 ] m^2"  interp_method=1  extrap_method=1  pr_dif=6e+05 Pa  reg_range=5e+04 Pa  C_d=0.7  x_0=0 m  A_leak=1e-12 m^2  lam_spec=1  B_lam=0.999  Re_cr=12
      settings: InternalSimscapePortConfiguration="{\"Bottom\":[],\"Left\":[{\"id\":\"C\",\"label\":\"C\",\"type\":\"input\"},{\"id\":\"A\",\"label\":\"A\",\"type\":\"foundation.hydraulic.hydraulic\"}],\"Right\":[{\"id\":\"B\",\"label\":\"B\",\"type\":\"foundation.hydraulic.hydraulic\"}],\"Top\":[]}"
  Signal Editor : SignalEditorBlockLib/Signal Editor  FileName=/Users/philip/Desktop/untitled folder/24hsiganls.mat  ActiveScenario=Scenario  ActiveSignal=00  IsBus=off  OutputBusObjectStr=Bus: BusObject  SampleTime=0  Interpolate=off  ZeroCross=off  OutputAfterFinalValue=Setting to zero  Unit=inherit  PreserveSignalName=on
  Simulink-PS Converter : nesl_utility/Simulink-PS Converter  PhysicalDomain=network_engine_domain  SubClassName=ps_input  LeftPortType=input  RightPortType=output  PseudoPeriodic=off  Frequencies=[]  NoiseDistribution=none  NoiseParameters=[]  Unit=1  AffineConversion=off  FilteringAndDerivatives=provide  SimscapeFilterOrder=1  InputFilterTimeConstant=0.001  UdotUserProvided=0
  Conn1 : PMIOPort  Side=Left
  Conn2 : PMIOPort  Port=2  Side=Right
  wires:
  Signal Editor/1 -> Simulink-PS Converter/1
  connections:
  Conn1/RConn1 -- Flow Control Valve/LConn2
  Flow Control Valve/RConn1 -- Conn2/RConn1
  Flow Control Valve/LConn1 -- Simulink-PS Converter/RConn1

== system combinedmodels/Subsystem1 ==
  Flow Control Valve : sh_lib/Valves/Flow Control Valves/Pressure-Compensated Flow Control Valve  Tag=Factory Generic  mdl_type=1  area_max=0.86e-4 m^2  opening_max=0.02 m  opening_tab="[  -0.002 0 0.005 0.015 ] m"  area_tab="[  1e-12 4e-12 1e-05 1.02e-05 ] m^2"  interp_method=1  extrap_method=1  pr_dif=6e+05 Pa  reg_range=5e+04 Pa  C_d=0.7  x_0=0 m  A_leak=1e-12 m^2  lam_spec=1  B_lam=0.999  Re_cr=12
      settings: InternalSimscapePortConfiguration="{\"Bottom\":[],\"Left\":[{\"id\":\"C\",\"label\":\"C\",\"type\":\"input\"},{\"id\":\"A\",\"label\":\"A\",\"type\":\"foundation.hydraulic.hydraulic\"}],\"Right\":[{\"id\":\"B\",\"label\":\"B\",\"type\":\"foundation.hydraulic.hydraulic\"}],\"Top\":[]}"
  Signal Editor : SignalEditorBlockLib/Signal Editor  FileName=/Users/philip/Desktop/untitled folder/24hsiganls.mat  ActiveScenario=Scenario  ActiveSignal=00  IsBus=off  OutputBusObjectStr=Bus: BusObject  SampleTime=0  Interpolate=off  ZeroCross=off  OutputAfterFinalValue=Setting to zero  Unit=inherit  PreserveSignalName=on
  Simulink-PS Converter : nesl_utility/Simulink-PS Converter  PhysicalDomain=network_engine_domain  SubClassName=ps_input  LeftPortType=input  RightPortType=output  PseudoPeriodic=off  Frequencies=[]  NoiseDistribution=none  NoiseParameters=[]  Unit=1  AffineConversion=off  FilteringAndDerivatives=provide  SimscapeFilterOrder=1  InputFilterTimeConstant=0.001  UdotUserProvided=0
  Conn2 : PMIOPort  Side=Right
  Conn1 : PMIOPort  Port=2  Side=Left
  wires:
  Signal Editor/1 -> Simulink-PS Converter/1
  connections:
  Conn2/RConn1 -- Flow Control Valve/LConn2
  Flow Control Valve/LConn1 -- Simulink-PS Converter/RConn1
  Flow Control Valve/RConn1 -- Conn1/RConn1

== system combinedmodels/Subsystem2 ==
  Flow Control Valve : sh_lib/Valves/Flow Control Valves/Pressure-Compensated Flow Control Valve  Tag=Factory Generic  mdl_type=1  area_max=0.86e-4 m^2  opening_max=0.02 m  opening_tab="[  -0.002 0 0.005 0.015 ] m"  area_tab="[  1e-12 4e-12 1e-05 1.02e-05 ] m^2"  interp_method=1  extrap_method=1  pr_dif=6e+05 Pa  reg_range=5e+04 Pa  C_d=0.7  x_0=0 m  A_leak=1e-12 m^2  lam_spec=1  B_lam=0.999  Re_cr=12
      settings: InternalSimscapePortConfiguration="{\"Bottom\":[],\"Left\":[{\"id\":\"C\",\"label\":\"C\",\"type\":\"input\"},{\"id\":\"A\",\"label\":\"A\",\"type\":\"foundation.hydraulic.hydraulic\"}],\"Right\":[{\"id\":\"B\",\"label\":\"B\",\"type\":\"foundation.hydraulic.hydraulic\"}],\"Top\":[]}"
  Signal Editor : SignalEditorBlockLib/Signal Editor  FileName=/Users/philip/Desktop/untitled folder/24hsiganls.mat  ActiveScenario=Scenario  ActiveSignal=00  IsBus=off  OutputBusObjectStr=Bus: BusObject  SampleTime=0  Interpolate=off  ZeroCross=off  OutputAfterFinalValue=Setting to zero  Unit=inherit  PreserveSignalName=on
  Simulink-PS Converter : nesl_utility/Simulink-PS Converter  PhysicalDomain=network_engine_domain  SubClassName=ps_input  LeftPortType=input  RightPortType=output  PseudoPeriodic=off  Frequencies=[]  NoiseDistribution=none  NoiseParameters=[]  Unit=1  AffineConversion=off  FilteringAndDerivatives=provide  SimscapeFilterOrder=1  InputFilterTimeConstant=0.001  UdotUserProvided=0
  Conn1 : PMIOPort  Side=Left
  Conn2 : PMIOPort  Port=2  Side=Right
  wires:
  Signal Editor/1 -> Simulink-PS Converter/1
  connections:
  Conn1/RConn1 -- Flow Control Valve/LConn2
  Conn2/RConn1 -- Flow Control Valve/RConn1
  Flow Control Valve/LConn1 -- Simulink-PS Converter/RConn1

== system combinedmodels/Volume T1 ==
  Reservoir : nesl_utility/PS-Simulink Converter  PhysicalDomain=network_engine_domain  SubClassName=ps_output  LeftPortType=input  RightPortType=output  PseudoPeriodic=off  Frequencies=[]  VectorFormat=1-D array  Unit=1  AffineConversion=off
  V : PMIOPort  Side=Left
  tag scope: V_S1=global
  wires:
  Reservoir/1 -> [V_S1]
  connections:
  Reservoir/LConn1 -- V/RConn1

== system combinedmodels/Volume T2 ==
  Storage Tank 1 : nesl_utility/PS-Simulink Converter  PhysicalDomain=network_engine_domain  SubClassName=ps_output  LeftPortType=input  RightPortType=output  PseudoPeriodic=off  Frequencies=[]  VectorFormat=1-D array  Unit=1  AffineConversion=off
  V : PMIOPort  Side=Left
  tag scope: V_S2=global
  wires:
  Storage Tank 1/1 -> [V_S2]
  connections:
  Storage Tank 1/LConn1 -- V/RConn1

== system combinedmodels/Volume T3 ==
  Storage Tank 2 : nesl_utility/PS-Simulink Converter  PhysicalDomain=network_engine_domain  SubClassName=ps_output  LeftPortType=input  RightPortType=output  PseudoPeriodic=off  Frequencies=[]  VectorFormat=1-D array  Unit=1  AffineConversion=off
  V : PMIOPort  Side=Left
  tag scope: V_S3=global
  wires:
  Storage Tank 2/1 -> [V_S3]
  connections:
  Storage Tank 2/LConn1 -- V/RConn1

== system combinedmodels/Volume T4 ==
  Output Tank 1 : nesl_utility/PS-Simulink Converter  PhysicalDomain=network_engine_domain  SubClassName=ps_output  LeftPortType=input  RightPortType=output  PseudoPeriodic=off  Frequencies=[]  VectorFormat=1-D array  Unit=1  AffineConversion=off
  V : PMIOPort  Side=Left
  tag scope: V_S4=global
  wires:
  Output Tank 1/1 -> [V_S4]
  connections:
  Output Tank 1/LConn1 -- V/RConn1

== system combinedmodels/Volume T5 ==
  Output Tank 2 : nesl_utility/PS-Simulink Converter  PhysicalDomain=network_engine_domain  SubClassName=ps_output  LeftPortType=input  RightPortType=output  PseudoPeriodic=off  Frequencies=[]  VectorFormat=1-D array  Unit=1  AffineConversion=off
  V : PMIOPort  Side=Left
  tag scope: V_S5=global
  wires:
  Output Tank 2/1 -> [V_S5]
  connections:
  Output Tank 2/LConn1 -- V/RConn1

== system combinedmodels/Volume T6 ==
  Output Tank 3 : nesl_utility/PS-Simulink Converter  PhysicalDomain=network_engine_domain  SubClassName=ps_output  LeftPortType=input  RightPortType=output  PseudoPeriodic=off  Frequencies=[]  VectorFormat=1-D array  Unit=1  AffineConversion=off
  V : PMIOPort  Side=Left
  tag scope: V_S6=global
  wires:
  Output Tank 3/1 -> [V_S6]
  connections:
  Output Tank 3/LConn1 -- V/RConn1

== system combinedmodels/Bus_10/VI Recorder13 ==
  Vrec : Inport
  Irec : Inport  Port=2
  tag scope: I9to10=global, V9to10=global
  wires:
  Vrec/1 -> [V9to10]
  Irec/1 -> [I9to10]

== system combinedmodels/Bus_11/VI Recorder14 ==
  Vrec : Inport
  Irec : Inport  Port=2
  tag scope: I10to11=global, V10to11=global
  wires:
  Vrec/1 -> [V10to11]
  Irec/1 -> [I10to11]

== system combinedmodels/Bus_12/VI Recorder15 ==
  Vrec : Inport
  Irec : Inport  Port=2
  tag scope: I11to12=global, V11to12=global
  wires:
  Vrec/1 -> [V11to12]
  Irec/1 -> [I11to12]

== system combinedmodels/Bus_13/VI Recorder16 ==
  Vrec : Inport
  Irec : Inport  Port=2
  tag scope: I12to13=global, V12to13=global
  wires:
  Vrec/1 -> [V12to13]
  Irec/1 -> [I12to13]

== system combinedmodels/Bus_14/VI Recorder17 ==
  Vrec : Inport
  Irec : Inport  Port=2
  tag scope: I13to14=global, V13to14=global
  wires:
  Vrec/1 -> [V13to14]
  Irec/1 -> [I13to14]

== system combinedmodels/Bus_15/VI Recorder18 ==
  Vrec : Inport
  Irec : Inport  Port=2
  tag scope: I14to15=global, V14to15=global
  wires:
  Vrec/1 -> [V14to15]
  Irec/1 -> [I14to15]

== system combinedmodels/Bus_16/VI Recorder19 ==
  Vrec : Inport
  Irec : Inport  Port=2
  tag scope: I15to16=global, V15to16=global
  wires:
  Vrec/1 -> [V15to16]
  Irec/1 -> [I15to16]

== system combinedmodels/Bus_17/VI Recorder20 ==
  Vrec : Inport
  Irec : Inport  Port=2
  tag scope: I16to17=global, V16to17=global
  wires:
  Vrec/1 -> [V16to17]
  Irec/1 -> [I16to17]

== system combinedmodels/Bus_18/VI Recorder21 ==
  Vrec : Inport
  Irec : Inport  Port=2
  tag scope: I17to18=global, V17to18=global
  wires:
  Vrec/1 -> [V17to18]
  Irec/1 -> [I17to18]

== system combinedmodels/Bus_19/VI Recorder ==
  Vrec : Inport
  Irec : Inport  Port=2
  tag scope: I2to19=global, V2to19=global
  wires:
  Vrec/1 -> [V2to19]
  Irec/1 -> [I2to19]

== system combinedmodels/Bus_2/VI Recorder5 ==
  Vrec : Inport
  Irec : Inport  Port=2
  tag scope: I1to2=global, V1to2=global
  wires:
  Vrec/1 -> [V1to2]
  Irec/1 -> [I1to2]

== system combinedmodels/Bus_20/VI Recorder1 ==
  Vrec : Inport
  Irec : Inport  Port=2
  tag scope: I19to20=global, V19to20=global
  wires:
  Vrec/1 -> [V19to20]
  Irec/1 -> [I19to20]

== system combinedmodels/Bus_21/VI Recorder2 ==
  Vrec : Inport
  Irec : Inport  Port=2
  tag scope: I20to21=global, V20to21=global
  wires:
  Vrec/1 -> [V20to21]
  Irec/1 -> [I20to21]

== system combinedmodels/Bus_22/VI Recorder3 ==
  Vrec : Inport
  Irec : Inport  Port=2
  tag scope: I21to22=global, V21to22=global
  wires:
  Vrec/1 -> [V21to22]
  Irec/1 -> [I21to22]

== system combinedmodels/Bus_23/VI Recorder32 ==
  Vrec : Inport
  Irec : Inport  Port=2
  tag scope: I3to23=global, V3to23=global
  wires:
  Vrec/1 -> [V3to23]
  Irec/1 -> [I3to23]

== system combinedmodels/Bus_24/VI Recorder31 ==
  Vrec : Inport
  Irec : Inport  Port=2
  tag scope: I23to24=global, V23to24=global
  wires:
  Vrec/1 -> [V23to24]
  Irec/1 -> [I23to24]

== system combinedmodels/Bus_25/VI Recorder30 ==
  Vrec : Inport
  Irec : Inport  Port=2
  tag scope: I24to25=global, V24to25=global
  wires:
  Vrec/1 -> [V24to25]
  Irec/1 -> [I24to25]

== system combinedmodels/Bus_26/VI Recorder22 ==
  Vrec : Inport
  Irec : Inport  Port=2
  tag scope: I6to26=global, V6to26=global
  wires:
  Vrec/1 -> [V6to26]
  Irec/1 -> [I6to26]

== system combinedmodels/Bus_27/VI Recorder23 ==
  Vrec : Inport
  Irec : Inport  Port=2
  tag scope: I26to27=global, V26to27=global
  wires:
  Vrec/1 -> [V26to27]
  Irec/1 -> [I26to27]

== system combinedmodels/Bus_28/VI Recorder24 ==
  Vrec : Inport
  Irec : Inport  Port=2
  tag scope: I27to28=global, V27to28=global
  wires:
  Vrec/1 -> [V27to28]
  Irec/1 -> [I27to28]

== system combinedmodels/Bus_29/VI Recorder25 ==
  Vrec : Inport
  Irec : Inport  Port=2
  tag scope: I28to29=global, V28to29=global
  wires:
  Vrec/1 -> [V28to29]
  Irec/1 -> [I28to29]

== system combinedmodels/Bus_3/VI Recorder6 ==
  Vrec : Inport
  Irec : Inport  Port=2
  tag scope: I2to3=global, V2to3=global
  wires:
  Vrec/1 -> [V2to3]
  Irec/1 -> [I2to3]

== system combinedmodels/Bus_30/VI Recorder26 ==
  Vrec : Inport
  Irec : Inport  Port=2
  tag scope: I29to30=global, V29to30=global
  wires:
  Vrec/1 -> [V29to30]
  Irec/1 -> [I29to30]

== system combinedmodels/Bus_31/VI Recorder27 ==
  Vrec : Inport
  Irec : Inport  Port=2
  tag scope: I30to31=global, V30to31=global
  wires:
  Vrec/1 -> [V30to31]
  Irec/1 -> [I30to31]

== system combinedmodels/Bus_32/VI Recorder28 ==
  Vrec : Inport
  Irec : Inport  Port=2
  tag scope: I31to32=global, V31to32=global
  wires:
  Vrec/1 -> [V31to32]
  Irec/1 -> [I31to32]

== system combinedmodels/Bus_33/VI Recorder29 ==
  Vrec : Inport
  Irec : Inport  Port=2
  tag scope: I32to33=global, V32to33=global
  wires:
  Vrec/1 -> [V32to33]
  Irec/1 -> [I32to33]

== system combinedmodels/Bus_4/VI Recorder7 ==
  Vrec : Inport
  Irec : Inport  Port=2
  tag scope: I3to4=global, V3to4=global
  wires:
  Vrec/1 -> [V3to4]
  Irec/1 -> [I3to4]

== system combinedmodels/Bus_5/VI Recorder8 ==
  Vrec : Inport
  Irec : Inport  Port=2
  tag scope: I4to5=global, V4to5=global
  wires:
  Vrec/1 -> [V4to5]
  Irec/1 -> [I4to5]

== system combinedmodels/Bus_6/VI Recorder9 ==
  Vrec : Inport
  Irec : Inport  Port=2
  tag scope: I5to6=global, V5to6=global
  wires:
  Vrec/1 -> [V5to6]
  Irec/1 -> [I5to6]

== system combinedmodels/Bus_7/VI Recorder10 ==
  Vrec : Inport
  Irec : Inport  Port=2
  tag scope: I6to7=global, V6to7=global
  wires:
  Vrec/1 -> [V6to7]
  Irec/1 -> [I6to7]

== system combinedmodels/Bus_8/VI Recorder11 ==
  Vrec : Inport
  Irec : Inport  Port=2
  tag scope: I7to8=global, V7to8=global
  wires:
  Vrec/1 -> [V7to8]
  Irec/1 -> [I7to8]

== system combinedmodels/Bus_9/VI Recorder12 ==
  Vrec : Inport
  Irec : Inport  Port=2
  tag scope: I8to9=global, V8to9=global
  wires:
  Vrec/1 -> [V8to9]
  Irec/1 -> [I8to9]
